simulink model "Versuch_2_Hybridmodell_Vorlage"  (R2024a)
settings: Solver=ode1  StartTime=0.0  StopTime=7645  FixedStep=0.1  RelTol=1e-3  EnableMultiTasking=on
values from neighbouring files (symbols this model uses):
  A = 1    [init.m]
  Cn = 30    [init.m]
  Cw = 1.1    [init.m]
  fr = 0.02    [init.m]
  g = 9.81    [init.m]
  i1 = 74/9    (= 8.22222222222)    [init.m]
  i2 = 58/10    (= 5.8)    [init.m]
  Jachse_mitte = 0.003    [init.m]
  Jachse_unten = 0.052    [init.m]
  Jmotor = 0.001    [init.m]
  Jrad = 0.2    [init.m]
  Kp = 4000    [init.m]
  m = 455    [init.m]
  rho = 1.2    [init.m]
  rR = 0.2434    [init.m]
  Tn = 200    [init.m]
  Un = 48    [init.m]
undefined symbols (not defined in the file or in its folder): altitude2_lookup, distance2_lookup, etaGe, etaInvMG2, gradient_distance_lookup, gradient_lookup, kennmg2, M_etaGe, nMG2, t_ece, v_ece
settings Model: Creator=roustiam  LastModifiedBy=Nico Hörter
settings SolverCC: AlgebraicLoopSolver=TrustRegion
settings DataIOCC: LimitDataPoints=on  SaveFormat=Array  SignalLoggingSaveFormat=ModelDataLogs  ReturnWorkspaceOutputs=off  SignalLoggingName=sigsOut
settings OptimizationCC: BlockReduction=off  BooleanDataType=off  ExpressionDepthLimit=2147483647  InitFltsAndDblsToZero=on  LifeSpan=inf
settings DebuggingCC: SaveWithParameterizedLinksMsg=none  UnderspecifiedInitializationDetection=Classic  MergeDetectMultiDrivingBlocksExec=none  SignalResolutionControl=TryResolveAllWithWarning  MultiTaskDSMMsg=warning  MultiTaskCondExecSysMsg=none  FcnCallInpInsideContextMsg=warning  UnconnectedInputMsg=warning  UnconnectedOutputMsg=warning  UnconnectedLineMsg=warning  StateNameClashWarn=warning  SFUnexpectedBacktrackingDiag=warning  SFNoUnconditionalDefaultTransitionDiag=warning  ArithmeticOperatorsInVariantConditions=warning
settings HardwareCC: ProdBitPerPointer=32  ProdBitPerSizeT=32  ProdBitPerPtrDiffT=32  ProdLargestAtomicFloat=None  ProdIntDivRoundTo=Undefined  ProdEndianess=Unspecified  ProdWordSize=32  ProdHWDeviceType=32-bit Generic  TargetUnknown=on
settings ModelReferenceCC: EnableRefExpFcnMdlSchedulingChecks=on  PropagateSignalLabelsOutOfModel=off
settings SFSimCC: SimUseLocalCustomCode=off  CustomCodeUndefinedFunction=UseInterfaceOnly
settings RTWCC: RTWUseLocalCustomCode=off  GPUComputeCapability=3.5
settings CodeAppCC: StateflowObjectComments=on
settings GRTTargetCC: TargetFcnLib=ansi_tfl_tmw.mat  TargetLangStandard=C89/C90 (ANSI)  CombineOutputUpdateFcns=off  GRTInterface=on
settings ConfigComp: CovMetricSettings=dw  CovSaveCumulativeToWorkspaceVar=on  CovSaveSingleToWorkspaceVar=on  CovExternalEMLEnable=off

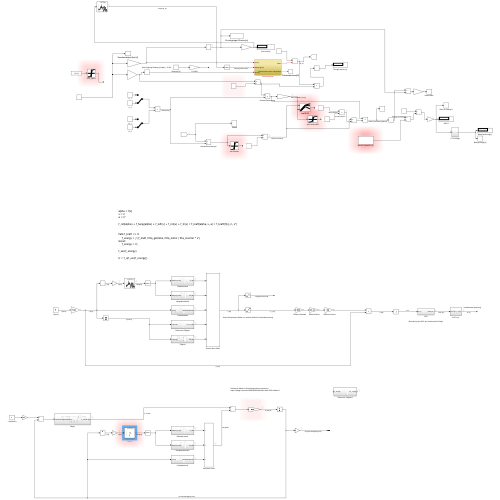
[thumbnail: Simulink's stored preview of the top-level diagram]
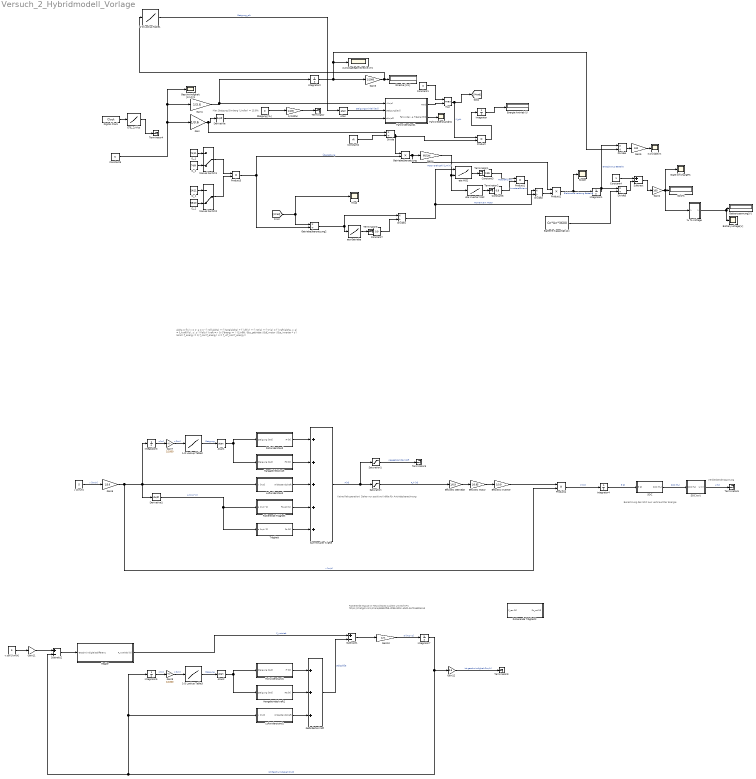
== system Versuch_2_Hybridmodell_Vorlage ==
  note: Rotierende Masse in Gewichtsequivalent umrechnen:
      | https://chatgpt.com/share/68552f58-d298-800c-abd2-5a7b1e80aca3
  note: Berechnung des SOC aus verbrauchter Energie
  note: alpha = f(s)
      | v = s'
      | a = s''
      |
      | f_roll(alpha) + f_hang(alpha) + f_luft(v) + f_rot(a) + f_tr(a) = f_kraft(alpha, v, a) = f_kraft(f(s), s', s'')
      |
      | Falls f_kraft => 0:
      | f_energy = ∫ (f_kraft / Eta_getriebe / Eta_motor / Eta_inverter * s')
      | Sonst:
      | f_energy = 0;
      |
      | f_soc(f_energy)
      |
      | U = f_u(f_soc(f_energy))
  note: Verbleibende Spannung
  note: Keine Rekuperation! Daher nur positive Kräfte für Antriebsberechnung
  note: Max Steigung Dimberg (Lindlar) = 15.8%
  " Mrad" : Scope
  % To Voltage : Subsystem
  1-D Lookup Table1 : Lookup_n-D  NumberOfTableDimensions=1  BreakpointsForDimension1=distance2_lookup  Table=altitude2_lookup  ExtrapMethod=Clip  InternalRulePriority=Speed  RndMeth=Simplest
  1-D Lookup Table2 : Lookup_n-D  NumberOfTableDimensions=1  BreakpointsForDimension1=distance2_lookup  Table=altitude2_lookup  ExtrapMethod=Clip  InternalRulePriority=Speed  RndMeth=Simplest
  1-D Lookup Table3 : Lookup_n-D  NumberOfTableDimensions=1  BreakpointsForDimension1=gradient_distance_lookup  Table=gradient_lookup  ExtrapMethod=Clip  InternalRulePriority=Speed  RndMeth=Simplest
  1/(100%) : Gain  Gain=1/100
  Atan : Trigonometry  Operator=atan
  Atan1 : Trigonometry  Operator=atan
  Atan2 : Trigonometry  Operator=atan
  Batterie Kapazität [J]x : Constant  Value=Cn*Un*3600
  Batterispannung[V] : Display
  Batteryvoltage[V] : Scope
  Constant1 : Constant  Value=0
  Constant2 : Constant  Value=rR
  Constant3 : Constant  Value=0.85
  Constant4 : Constant
  Constant5 : Constant  Value=5
  Constant6 : Constant  Value=0.9
  Constant7 : Constant  Value=0.9
  Derivative : Derivative
  Derivative1 : Derivative
  Digital Clock : DigitalClock  SampleTime=0.1
  Divide{,1..4} (5 alike) : Product  Inputs=*/
  ETE_Zyklus : Lookup  InputValues=t_ece  Table=v_ece  SaturateOnIntegerOverflow=off
  Effizienz Getriebe : Gain  Gain=1/0.9
  Effizienz Inverter : Gain  Gain=1/0.9
  Effizienz Motor : Gain  Gain=1/0.85
  Energie Antrieb (J) : Display
  Fahrwiderstand1 : Subsystem
  Fahrwiederstand[N] : Scope
  Gain{,1,6,11} (4 alike) : Gain  Gain=1/3.6
  Gain10 : Gain  Gain=1/m
  Gain12 : Gain  Gain=3.6
  Gain2 : Gain  Gain=100
  Gain3 : Gain  Gain=1/1000
  Gain4 : Gain  Gain=60/2/pi
  Gain5 : Gain  Gain=100
  Gain7 : Gain  Gain=1/1000
  Gain9 : Gain  Gain=1/1000
  Geforderte Kraft : Sum  Inputs=+++
  Geschwindigkeit [km/h]1 : Scope
  Getriebeübersetzung : Product
  Getriebeübersetzung2 : Product  Inputs=*/
  Hangabtriebskraft : Subsystem
  Hangabtriebskraft1 : Subsystem
  I1_1 : Constant  Value=74/11
  I1_2 : Constant  Value=74/9
  I2_1 : Constant  Value=24/11
  I2_2 : Constant  Value=58/10
  Integrator{,1..5,7} (7 alike) : Integrator
  Kwh/100Km : Scope
  Luftwiderstand : Subsystem
  Luftwiderstand1 : Subsystem
  Manual Switch1 : ManualSwitch  CurrentSetting=0
  Manual Switch2 : ManualSwitch  CurrentSetting=0
  Max : MinMax  Function=max  Inputs=2
  Product{,1..4} (5 alike) : Product
  Regler : Subsystem
  Rollwiderstand : Subsystem
  Rollwiderstand1 : Subsystem
  Rotierende Trägheit : Subsystem
  Rotierende Trägheit2 : Subsystem
  SOC : Subsystem
  SOC to U : Subsystem
  SOC% : Display
  Saturation : Saturate  UpperLimit=inf  LowerLimit=0
  Saturation1 : Saturate  UpperLimit=0  LowerLimit=-inf
  Scope : Scope
  State Of Charge% : Scope
  Steigung [%] : Constant  Value=0
  Strecke [km] : Display
  Subtract : Sum  Inputs=+-
  Subtract1 : Sum  Inputs=+-
  Subtract2 : Sum  Inputs=+-
  Summe aller Kräfte : Sum  Inputs=+++++
  Terminator{,1..6,9} (8 alike) : Terminator
  Trägheit : Subsystem
  Zurückgelegte Strecke [m] : Scope
  eta Getriebe : Lookup  InputValues=M_etaGe  Table=etaGe  SaturateOnIntegerOverflow=off
  eta Inverter MG2 : Lookup  InputValues=nMG2  Table=etaInvMG2  SaturateOnIntegerOverflow=off
  eta MG2 : Lookup2D  RowIndex=mmg2  ColumnIndex=nmg2  Table=kennmg2
  v [km/h] : Constant  Value=5
  v soll [km/h] : Constant  Value=5
  wires:
  Digital Clock/1 -> ETE_Zyklus/1
  ETE_Zyklus/1 -> Terminator4/1
  [Mrad] -> Getriebeübersetzung2/1, " Mrad"/1
  Constant5/1 -> Geschwindigkeit [km/h]1/1, Gain1/1, Gain/1
  Derivative/1 -> Fahrwiderstand1/3(a[m/s2])
  Gain/1 -> Divide/1, Derivative/1
  Gain1/1 -> Integrator2/1, Fahrwiderstand1/1(v[m/s])
  Integrator/1 -> Energie Antrieb (J)/1
  Fahrwiderstand1/2(Fahrwiderstand (Ohne Trägheit)[N]) -> Fahrwiederstand[N]/1
  Constant1/1 -> Max/1
  Fahrwiderstand1/1(Mrad) -> Max/2
  Max/1 -> Product/1, [Mrad]  "M_alt"
  Divide/1 -> Getriebeübersetzung/1, Product/2
  Constant2/1 -> Divide/2
  Product/1 -> Integrator/1
  Getriebeübersetzung2/1 -> Divide1/1, eta Getriebe/1
  Divide1/1 -> Divide2/1, eta MG2/1  "Moment am Motor"
  Gain4/1 -> eta Inverter MG2/1, eta MG2/2  "Motor Drehzahl [1/min]"
  Product1/1 -> Divide2/2
  Getriebeübersetzung/1 -> Gain4/1, Product2/1
  Divide2/1 -> Product2/2
  Product2/1 -> Scope/1, Integrator1/1  "Elektrische Leistung Batterie"
  Integrator1/1 -> Divide4/1, Divide3/1  "Energie aus Batterie"
  Constant4/1 -> Subtract/1
  Divide3/1 -> Subtract/2
  Subtract/1 -> Gain2/1
  Batterie Kapazität [J]x/1 -> Divide3/2
  Integrator2/1 -> Zurückgelegte Strecke [m]/1, Divide4/2, Gain3/1
  eta MG2/1 -> Terminator1/1
  Constant3/1 -> Product1/1  "Motoreffizienz"
  eta Inverter MG2/1 -> Terminator2/1
  Constant6/1 -> Product1/2  "Invertereffizienz"
  eta Getriebe/1 -> Terminator3/1
  Constant7/1 -> Divide1/2
  Gain2/1 -> % To Voltage/1(In1), State Of Charge%/1, SOC%/1
  Steigung [%]/1 -> 1/(100%)/1
  Atan/1 -> Fahrwiderstand1/2(Steigung[rad])  "Steigungswinkel [rad]"
  Product3/1 -> Getriebeübersetzung2/2, Getriebeübersetzung/2  "Übersetzung"
  Gain3/1 -> 1-D Lookup Table1/1, Strecke [km]/1
  I2_1/1 -> Manual Switch2/1
  I2_2/1 -> Manual Switch2/2
  I1_1/1 -> Manual Switch1/1
  I1_2/1 -> Manual Switch1/2
  Manual Switch1/1 -> Product3/1
  Manual Switch2/1 -> Product3/2
  % To Voltage/1(Out1) -> Batterispannung[V]/1, Batteryvoltage[V]/1
  Divide4/1 -> Gain5/1
  Gain5/1 -> Kwh/100Km/1
  1-D Lookup Table1/1 -> Atan/1  "Steigung_alt"
  1/(100%)/1 -> Terminator/1
  v [km/h]/1 -> Gain6/1  "v [km/h]"
  Integrator3/1 -> Gain7/1  "s [m]"
  Derivative1/1 -> Trägheit/1(a [m/s^2]), Rotierende Trägheit/1(a [m/s^2])  "a [m/s^2]"
  Rotierende Trägheit/1(Ftr_rot [N]) -> Summe aller Kräfte/4
  Trägheit/1(Ftr [N]) -> Summe aller Kräfte/5
  Luftwiderstand/1(Widerstandskraft) -> Summe aller Kräfte/3
  Hangabtriebskraft/1(Fst [N]) -> Summe aller Kräfte/2
  Rollwiderstand/1(Fr [N]) -> Summe aller Kräfte/1
  Summe aller Kräfte/1 -> Saturation1/1, Saturation/1  "F [N]"
  Saturation1/1 -> Terminator5/1  "weggebremste Kraft"
  Saturation/1 -> Effizienz Getriebe/1  "F_+ [N]"
  Effizienz Getriebe/1 -> Effizienz Motor/1
  Effizienz Motor/1 -> Effizienz Inverter/1
  Gain6/1 -> Product4/2, Derivative1/1, Luftwiderstand/1(v [m/s]), Integrator3/1  "v [m/s]"
  Effizienz Inverter/1 -> Product4/1
  Product4/1 -> Integrator4/1  "P [W]"
  Integrator4/1 -> SOC/1(E [J])  "E [J]"
  SOC/1(SOC [%]) -> SOC to U/1(SOC [%])  "SOC [%]"
  SOC to U/1(U [V]) -> Terminator6/1  "U [V]"
  1-D Lookup Table2/1 -> Atan1/1  "Steigung"
  Atan1/1 -> Rollwiderstand/1(Steigung [rad]), Hangabtriebskraft/1(Steigung [rad])
  Gain7/1 -> 1-D Lookup Table2/1  "s [km]"
  Atan2/1 -> Rollwiderstand1/1(Steigung [rad]), Hangabtriebskraft1/1(Steigung [rad])
  1-D Lookup Table3/1 -> Atan2/1  "Steigung"
  Gain9/1 -> 1-D Lookup Table3/1  "s [km]"
  Integrator5/1 -> Gain9/1  "s [m]"
  Rollwiderstand1/1(Fr [N]) -> Geforderte Kraft/1
  Hangabtriebskraft1/1(Fst [N]) -> Geforderte Kraft/2
  Luftwiderstand1/1(Widerstandskraft) -> Geforderte Kraft/3
  Gain10/1 -> Integrator7/1  "a [m/s^2]"
  Integrator7/1 -> Gain12/1, Integrator5/1, Luftwiderstand1/1(v [m/s]), Subtract2/2  "Ist Geschwindigkeit [m/s]"
  Geforderte Kraft/1 -> Subtract1/2  "Störgröße"
  Regler/1(F_vortrieb [N]) -> Subtract1/1  "F_vortrieb"
  Subtract1/1 -> Gain10/1
  v soll [km/h]/1 -> Gain11/1
  Gain11/1 -> Subtract2/1
  Subtract2/1 -> Regler/1(Geschwindigkeitsdifferenz)
  Gain12/1 -> Terminator9/1  "Ist geschwindigkeit [km/h]"

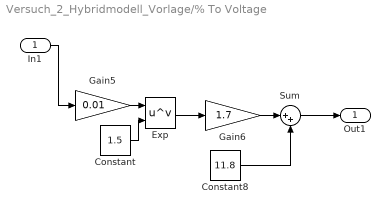
== system Versuch_2_Hybridmodell_Vorlage/% To Voltage ==
  In1 : Inport
  Constant : Constant  Value=1.5
  Constant8 : Constant  Value=11.8
  Exp : Math  Operator=pow
  Gain5 : Gain  Gain=0.01
  Gain6 : Gain  Gain=1.7
  Sum : Sum  Inputs=|++
  Out1 : Outport
  wires:
  Constant/1 -> Exp/2
  Gain6/1 -> Sum/1
  Exp/1 -> Gain6/1
  Gain5/1 -> Exp/1
  Constant8/1 -> Sum/2
  In1/1 -> Gain5/1
  Sum/1 -> Out1/1

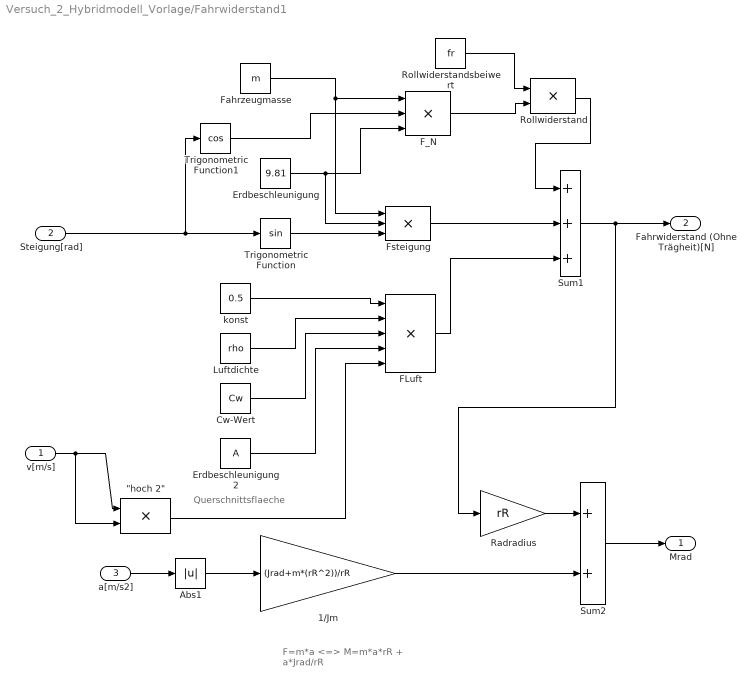
== system Versuch_2_Hybridmodell_Vorlage/Fahrwiderstand1 ==
  note: F=m*a <=> M=m*a*rR
      | +
      | a*Jrad/rR
  note: Querschnittsflaeche
  v[m/s] : Inport
  Steigung[rad] : Inport  Port=2
  a[m/s2] : Inport  Port=3
  "\"hoch 2\"" : Product  InputSameDT=on  RndMeth=Zero  SaturateOnIntegerOverflow=on  OutDataTypeStr=Inherit: Same as first input
  1/Jm : Gain  Gain=(Jrad+m*(rR^2))/rR
  Abs1 : Abs  SaturateOnIntegerOverflow=off
  Cw-Wert : Constant  Value=Cw
  "Erdbeschleunigung " : Constant  Value=9.81
  Erdbeschleunigung 2 : Constant  Value=A
  FLuft : Product  Inputs=5  InputSameDT=on  RndMeth=Zero  SaturateOnIntegerOverflow=on  OutDataTypeStr=Inherit: Same as first input
  F_N : Product  Inputs=3  InputSameDT=on  RndMeth=Zero  SaturateOnIntegerOverflow=on  OutDataTypeStr=Inherit: Same as first input
  Fahrzeugmasse : Constant  Value=m
  Fsteigung : Product  Inputs=3  InputSameDT=on  RndMeth=Zero  SaturateOnIntegerOverflow=on  OutDataTypeStr=Inherit: Same as first input
  Luftdichte : Constant  Value=rho
  Radradius : Gain  Gain=rR
  Rollwiderstand : Product  InputSameDT=on  RndMeth=Zero  SaturateOnIntegerOverflow=on  OutDataTypeStr=Inherit: Same as first input
  Rollwiderstandsbeiwert : Constant  Value=fr
  Sum1 : Sum  Inputs=+++  InputSameDT=on  SaturateOnIntegerOverflow=on  OutDataTypeStr=Inherit: Same as first input
  Sum2 : Sum  InputSameDT=on  SaturateOnIntegerOverflow=on  OutDataTypeStr=Inherit: Same as first input
  Trigonometric Function : Trigonometry
  Trigonometric Function1 : Trigonometry  Operator=cos
  konst : Constant  Value=0.5
  Mrad : Outport
  Fahrwiderstand (Ohne Trägheit)[N] : Outport  Port=2
  wires:
  Abs1/1 -> 1/Jm/1
  Sum2/1 -> Mrad/1
  Radradius/1 -> Sum2/1
  1/Jm/1 -> Sum2/2
  a[m/s2]/1 -> Abs1/1
  Rollwiderstandsbeiwert/1 -> Rollwiderstand/1
  Fahrzeugmasse/1 -> Fsteigung/1, F_N/1
  "Erdbeschleunigung "/1 -> F_N/3, Fsteigung/2
  Trigonometric Function/1 -> Fsteigung/3
  Steigung[rad]/1 -> Trigonometric Function/1, Trigonometric Function1/1
  "\"hoch 2\""/1 -> FLuft/5
  Erdbeschleunigung 2/1 -> FLuft/4
  Cw-Wert/1 -> FLuft/3
  Luftdichte/1 -> FLuft/2
  konst/1 -> FLuft/1
  F_N/1 -> Rollwiderstand/2
  Fsteigung/1 -> Sum1/2
  FLuft/1 -> Sum1/3
  Sum1/1 -> Radradius/1, Fahrwiderstand (Ohne Trägheit)[N]/1
  v[m/s]/1 -> "\"hoch 2\""/1, "\"hoch 2\""/2
  Trigonometric Function1/1 -> F_N/2
  Rollwiderstand/1 -> Sum1/1

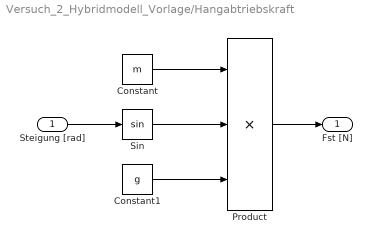
== system Versuch_2_Hybridmodell_Vorlage/Hangabtriebskraft ==
  Steigung [rad] : Inport
  Constant : Constant  Value=m
  Constant1 : Constant  Value=g
  Product : Product  Inputs=3
  Sin : Trigonometry
  Fst [N] : Outport
  wires:
  Product/1 -> Fst [N]/1
  Constant/1 -> Product/1
  Sin/1 -> Product/2
  Steigung [rad]/1 -> Sin/1
  Constant1/1 -> Product/3

== system Versuch_2_Hybridmodell_Vorlage/Hangabtriebskraft1 ==
  Steigung [rad] : Inport
  Constant : Constant  Value=m
  Constant1 : Constant  Value=g
  Product : Product  Inputs=3
  Sin : Trigonometry
  Fst [N] : Outport
  wires:
  Product/1 -> Fst [N]/1
  Constant/1 -> Product/1
  Sin/1 -> Product/2
  Steigung [rad]/1 -> Sin/1
  Constant1/1 -> Product/3

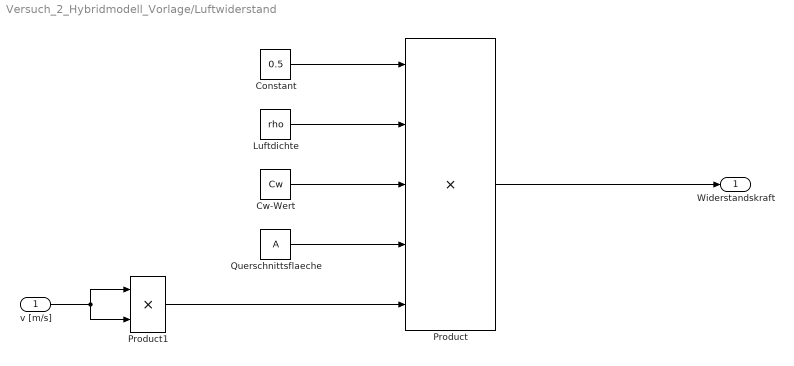
== system Versuch_2_Hybridmodell_Vorlage/Luftwiderstand ==
  v [m/s] : Inport
  Constant : Constant  Value=0.5
  Cw-Wert : Constant  Value=Cw
  Luftdichte : Constant  Value=rho
  Product : Product  Inputs=5
  Product1 : Product
  Querschnittsflaeche : Constant  Value=A
  Widerstandskraft : Outport
  wires:
  Querschnittsflaeche/1 -> Product/4
  Cw-Wert/1 -> Product/3
  Luftdichte/1 -> Product/2
  Constant/1 -> Product/1
  Product1/1 -> Product/5
  v [m/s]/1 -> Product1/1, Product1/2
  Product/1 -> Widerstandskraft/1

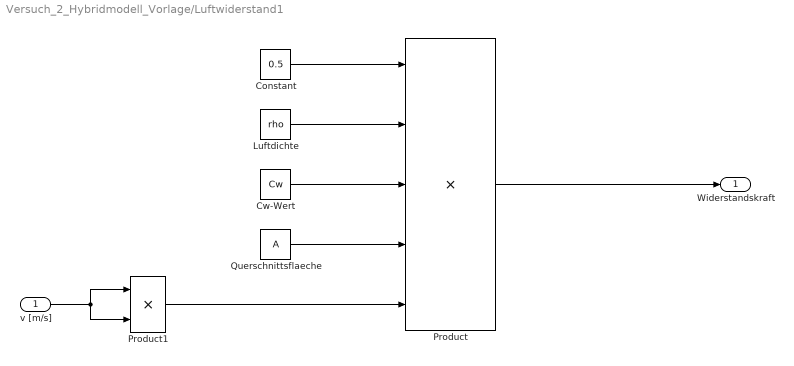
== system Versuch_2_Hybridmodell_Vorlage/Luftwiderstand1 ==
  v [m/s] : Inport
  Constant : Constant  Value=0.5
  Cw-Wert : Constant  Value=Cw
  Luftdichte : Constant  Value=rho
  Product : Product  Inputs=5
  Product1 : Product
  Querschnittsflaeche : Constant  Value=A
  Widerstandskraft : Outport
  wires:
  Querschnittsflaeche/1 -> Product/4
  Cw-Wert/1 -> Product/3
  Luftdichte/1 -> Product/2
  Constant/1 -> Product/1
  Product1/1 -> Product/5
  v [m/s]/1 -> Product1/1, Product1/2
  Product/1 -> Widerstandskraft/1

== system Versuch_2_Hybridmodell_Vorlage/Regler ==
  Geschwindigkeitsdifferenz : Inport
  Add : Sum
  Gain : Gain  Gain=1/Tn
  Integrator : Integrator
  Kp : Gain  Gain=Kp
  F_vortrieb [N] : Outport
  wires:
  Geschwindigkeitsdifferenz/1 -> Kp/1
  Add/1 -> F_vortrieb [N]/1
  Kp/1 -> Gain/1, Add/1
  Gain/1 -> Integrator/1
  Integrator/1 -> Add/2

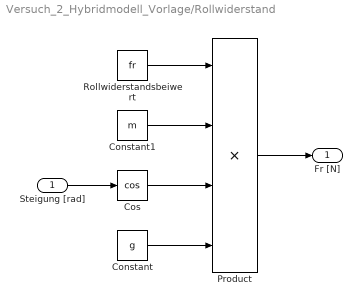
== system Versuch_2_Hybridmodell_Vorlage/Rollwiderstand ==
  Steigung [rad] : Inport
  Constant : Constant  Value=g
  Constant1 : Constant  Value=m
  Cos : Trigonometry  Operator=cos
  Product : Product  Inputs=4
  Rollwiderstandsbeiwert : Constant  Value=fr
  Fr [N] : Outport
  wires:
  Steigung [rad]/1 -> Cos/1
  Product/1 -> Fr [N]/1
  Constant/1 -> Product/4
  Cos/1 -> Product/3
  Constant1/1 -> Product/2
  Rollwiderstandsbeiwert/1 -> Product/1

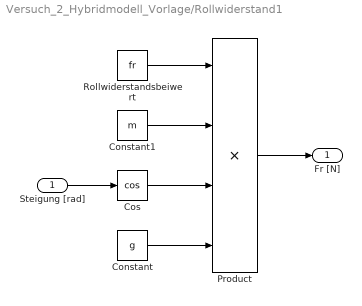
== system Versuch_2_Hybridmodell_Vorlage/Rollwiderstand1 ==
  Steigung [rad] : Inport
  Constant : Constant  Value=g
  Constant1 : Constant  Value=m
  Cos : Trigonometry  Operator=cos
  Product : Product  Inputs=4
  Rollwiderstandsbeiwert : Constant  Value=fr
  Fr [N] : Outport
  wires:
  Steigung [rad]/1 -> Cos/1
  Product/1 -> Fr [N]/1
  Constant/1 -> Product/4
  Cos/1 -> Product/3
  Constant1/1 -> Product/2
  Rollwiderstandsbeiwert/1 -> Product/1

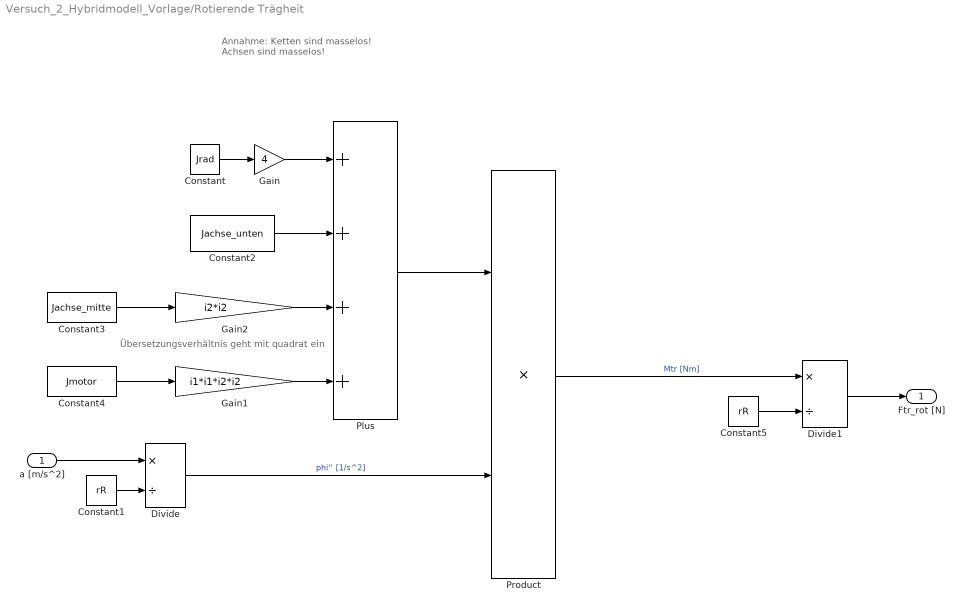
== system Versuch_2_Hybridmodell_Vorlage/Rotierende Trägheit ==
  note: Übersetzungsverhältnis geht mit quadrat ein
  note: Annahme: Ketten sind masselos!
      | Achsen sind masselos!
  a [m/s^2] : Inport
  Constant : Constant  Value=Jrad
  Constant1 : Constant  Value=rR
  Constant2 : Constant  Value=Jachse_unten
  Constant3 : Constant  Value=Jachse_mitte
  Constant4 : Constant  Value=Jmotor
  Constant5 : Constant  Value=rR
  Divide : Product  Inputs=*/  RndMeth=Zero  SaturateOnIntegerOverflow=on
  Divide1 : Product  Inputs=*/
  Gain : Gain  Gain=4
  Gain1 : Gain  Gain=i1*i1*i2*i2
  Gain2 : Gain  Gain=i2*i2
  Plus : Sum  Inputs=++++
  Product : Product
  Ftr_rot [N] : Outport
  wires:
  a [m/s^2]/1 -> Divide/1
  Constant1/1 -> Divide/2
  Divide/1 -> Product/2  "phi'' [1/s^2]"
  Constant/1 -> Gain/1
  Gain/1 -> Plus/1
  Constant2/1 -> Plus/2
  Plus/1 -> Product/1
  Product/1 -> Divide1/1  "Mtr [Nm]"
  Constant4/1 -> Gain1/1
  Constant3/1 -> Gain2/1
  Gain2/1 -> Plus/3
  Gain1/1 -> Plus/4
  Constant5/1 -> Divide1/2
  Divide1/1 -> Ftr_rot [N]/1

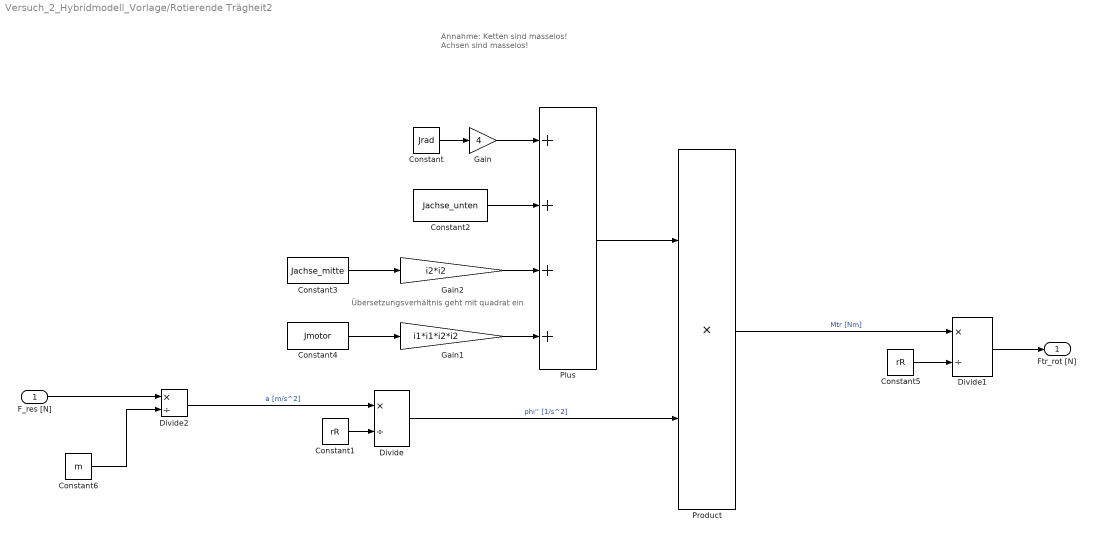
== system Versuch_2_Hybridmodell_Vorlage/Rotierende Trägheit2 ==
  note: Übersetzungsverhältnis geht mit quadrat ein
  note: Annahme: Ketten sind masselos!
      | Achsen sind masselos!
  F_res [N] : Inport
  Constant : Constant  Value=Jrad
  Constant1 : Constant  Value=rR
  Constant2 : Constant  Value=Jachse_unten
  Constant3 : Constant  Value=Jachse_mitte
  Constant4 : Constant  Value=Jmotor
  Constant5 : Constant  Value=rR
  Constant6 : Constant  Value=m
  Divide : Product  Inputs=*/  RndMeth=Zero  SaturateOnIntegerOverflow=on
  Divide1 : Product  Inputs=*/
  Divide2 : Product  Inputs=*/
  Gain : Gain  Gain=4
  Gain1 : Gain  Gain=i1*i1*i2*i2
  Gain2 : Gain  Gain=i2*i2
  Plus : Sum  Inputs=++++
  Product : Product
  Ftr_rot [N] : Outport
  wires:
  Constant1/1 -> Divide/2
  Divide/1 -> Product/2  "phi'' [1/s^2]"
  Constant/1 -> Gain/1
  Gain/1 -> Plus/1
  Constant2/1 -> Plus/2
  Plus/1 -> Product/1
  Product/1 -> Divide1/1  "Mtr [Nm]"
  Constant4/1 -> Gain1/1
  Constant3/1 -> Gain2/1
  Gain2/1 -> Plus/3
  Gain1/1 -> Plus/4
  Constant5/1 -> Divide1/2
  Divide1/1 -> Ftr_rot [N]/1
  Divide2/1 -> Divide/1  "a [m/s^2]"
  F_res [N]/1 -> Divide2/1
  Constant6/1 -> Divide2/2

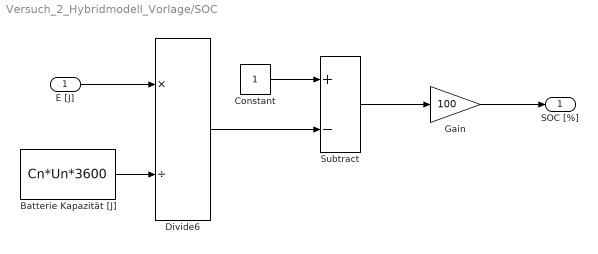
== system Versuch_2_Hybridmodell_Vorlage/SOC ==
  E [J] : Inport
  Batterie Kapazität [J] : Constant  Value=Cn*Un*3600
  Constant : Constant
  Divide6 : Product  Inputs=*/
  Gain : Gain  Gain=100
  Subtract : Sum  Inputs=+-
  SOC [%] : Outport
  wires:
  E [J]/1 -> Divide6/1
  Batterie Kapazität [J]/1 -> Divide6/2
  Divide6/1 -> Subtract/2
  Constant/1 -> Subtract/1
  Subtract/1 -> Gain/1
  Gain/1 -> SOC [%]/1

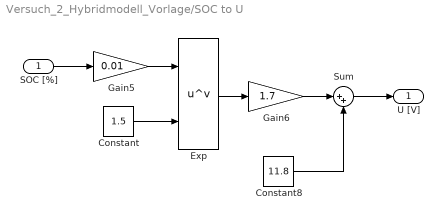
== system Versuch_2_Hybridmodell_Vorlage/SOC to U ==
  SOC [%] : Inport
  Constant : Constant  Value=1.5
  Constant8 : Constant  Value=11.8
  Exp : Math  Operator=pow
  Gain5 : Gain  Gain=0.01
  Gain6 : Gain  Gain=1.7
  Sum : Sum  Inputs=|++
  U [V] : Outport
  wires:
  Constant/1 -> Exp/2
  Gain6/1 -> Sum/1
  Exp/1 -> Gain6/1
  Gain5/1 -> Exp/1
  Constant8/1 -> Sum/2
  SOC [%]/1 -> Gain5/1
  Sum/1 -> U [V]/1

== system Versuch_2_Hybridmodell_Vorlage/Trägheit ==
  a [m/s^2] : Inport
  Masse : Constant  Value=m
  Product : Product
  Ftr [N] : Outport
  wires:
  a [m/s^2]/1 -> Product/2
  Product/1 -> Ftr [N]/1
  Masse/1 -> Product/1
